simulink model "Rover"  (Simulink 8.9)
settings: Solver=FixedStepAuto  StartTime=0.0  StopTime=100000  FixedStep=1/100  RelTol=1e-3
libraries: robotmobilelib x1, simulink x1
settings Model: Creator=Peter  LastModifiedBy=Peter
settings DataIOCC: LimitDataPoints=off  SaveFormat=Dataset  SignalLoggingSaveFormat=Dataset  ReturnWorkspaceOutputs=on
settings OptimizationCC: LifeSpan=auto
settings DebuggingCC: UnderspecifiedInitializationDetection=Simplified  MergeDetectMultiDrivingBlocksExec=error  FcnCallInpInsideContextMsg=error  StateNameClashWarn=none  SFUnexpectedBacktrackingDiag=error  SFNoUnconditionalDefaultTransitionDiag=error  SFExecutionAtInitializationDiag=warning
settings HardwareCC: ProdBitPerPointer=64  ProdBitPerSizeT=64  ProdBitPerPtrDiffT=64  ProdLargestAtomicFloat=Float  ProdIntDivRoundTo=Zero  ProdEndianess=LittleEndian  ProdWordSize=64  ProdHWDeviceType=Intel->x86-64 (Windows64)
settings ModelReferenceCC: PropagateSignalLabelsOutOfModel=on
settings SFSimCC: SimUseLocalCustomCode=on
settings RTWCC: RTWUseLocalCustomCode=on
settings GRTTargetCC: TargetLangStandard=C99 (ISO)  CombineOutputUpdateFcns=on  GRTInterface=off
settings ConfigComp: CovMetricSettings=dwe  CovHtmlReporting=off  CovSaveCumulativeToWorkspaceVar=off  CovSaveSingleToWorkspaceVar=off  CovExternalEMLEnable=on

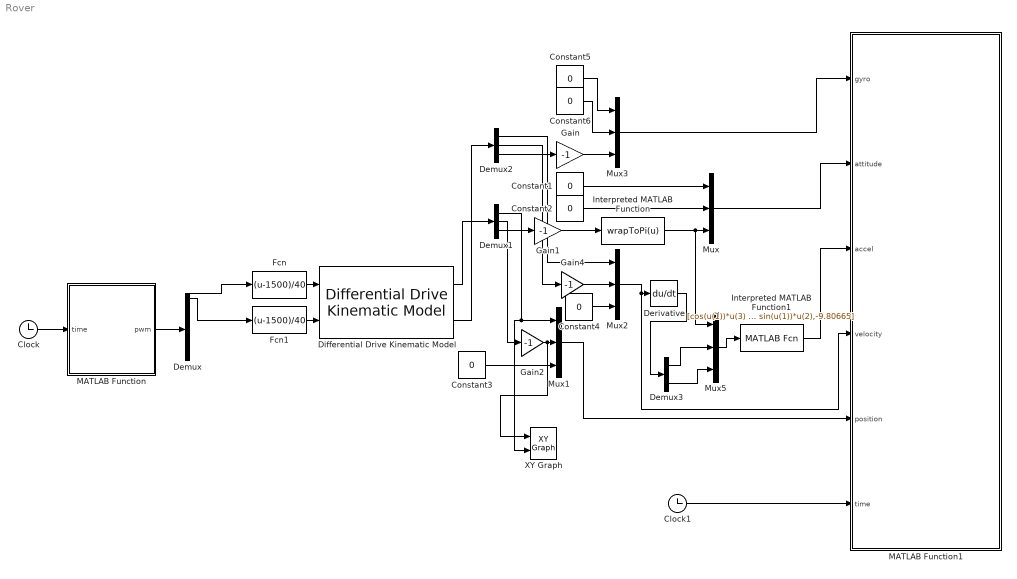
== system Rover ==
  Clock : Clock
  Clock1 : Clock
  Constant{1..6} (6 alike) : Constant  Value=0
  Demux : Demux  Outputs=16
  Demux1 : Demux  Outputs=3
  Demux2 : Demux  Outputs=3
  Demux3 : Demux  Outputs=2
  Derivative : Derivative
  Differential Drive Kinematic Model : robotmobilelib/Differential Drive Kinematic Model  VehicleInputs=Wheel Speeds  WheelRadius=0.16  WheelSpeedRange=[-100 100]  TrackWidth=0.2  InitialState=[0; 0; 0]  SimulateUsing=Interpreted execution
      settings: SourceProductBaseCode=RO
  Fcn : Fcn  Expr=(u-1500)/40
  Fcn1 : Fcn  Expr=(u-1500)/40
  Gain{,1..2,4} (4 alike) : Gain  Gain=-1
  Interpreted MATLAB Function : MATLABFcn  MATLABFcn=wrapToPi(u)
  Interpreted MATLAB Function1 : MATLABFcn  MATLABFcn=[cos(u(1))*u(3) + sin(u(1))*u(3),cos(u(1))*u(3) + sin(u(1))*u(2),-9.80665]
  MATLAB Function : MATLAB Function  TreatAsAtomicUnit=on
  MATLAB Function1 : MATLAB Function  TreatAsAtomicUnit=on
  Mux{,1..3,5} (5 alike) : Mux  Inputs=3
  XY Graph : simulink/Sinks/XY Graph  xmin=-inf  xmax=inf  ymin=-inf  ymax=inf  st=-1
  wires:
  Demux/2 -> Fcn1/1
  MATLAB Function/1(pwm) -> Demux/1
  Fcn/1 -> Differential Drive Kinematic Model/1
  Clock/1 -> MATLAB Function/1(time)
  Demux/1 -> Fcn/1
  Fcn1/1 -> Differential Drive Kinematic Model/2
  Clock1/1 -> MATLAB Function1/6(time)
  Differential Drive Kinematic Model/1 -> Demux1/1
  Demux1/3 -> Gain1/1
  Mux/1 -> MATLAB Function1/2(attitude)
  Constant1/1 -> Mux/1
  Constant2/1 -> Mux/2
  Mux1/1 -> MATLAB Function1/5(position)
  Demux1/2 -> Gain2/1
  Constant3/1 -> Mux1/3
  Differential Drive Kinematic Model/2 -> Demux2/1
  Constant4/1 -> Mux2/3
  Demux2/2 -> Gain4/1
  Demux2/1 -> Mux2/1
  Mux3/1 -> MATLAB Function1/1(gyro)
  Constant6/1 -> Mux3/2
  Constant5/1 -> Mux3/1
  Demux2/3 -> Gain/1
  Mux2/1 -> Derivative/1, MATLAB Function1/4(velocity)
  Gain/1 -> Mux3/3
  Gain1/1 -> Interpreted MATLAB Function/1
  Demux1/1 -> XY Graph/2, Mux1/1
  Gain2/1 -> XY Graph/1, Mux1/2
  Interpreted MATLAB Function/1 -> Mux5/1, Mux/3
  Gain4/1 -> Mux2/2
  Interpreted MATLAB Function1/1 -> MATLAB Function1/3(accel)
  Derivative/1 -> Demux3/1
  Demux3/2 -> Mux5/3
  Demux3/1 -> Mux5/2
  Mux5/1 -> Interpreted MATLAB Function1/1

== matlab function MATLAB Function1 ==
  data: gyro input double; attitude input double; accel input double; velocity input double; position input double; time input double
function fcn(gyro, attitude, accel, velocity, position, time)
coder.extrinsic('AP_send')
AP_send(gyro, attitude, accel, velocity, position, time)
end

== matlab function MATLAB Function ==
  data: pwm output double; time input double
function pwm  = fcn(time)
pwm = zeros(16,1);
coder.extrinsic('AP_receve')
pwm = AP_receve(time);
end
